simulink library "Lib_Turbo_Turbine_TMATS"  (R2012b)
settings: Solver=ode45  StartTime=0.0  StopTime=10.0  RelTol=1e-3
Description:
  | Thomas Modules
settings Model: Creator=jwchapm2  LastModifiedBy=jwchapm2

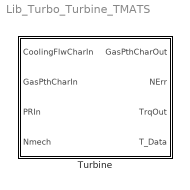
== system Lib_Turbo_Turbine_TMATS ==
  Turbine : Subsystem  mask(T-MATS: Turbine Library Block){X_T_PRVec_M=[ 3.000  8.000], Y_T_NcVec_M=[60 80  110], T_T_Map_WcArray_M=[0 0;0 0; 0 0], T_T_Map_EffArray_M=[0 0; 0 0; 0 0], s_T_Nc_M=0.0243, s_T_PR_M=0.9736, s_T_Wc_M=0.4504, s_T_Eff_M=0.9984, CFlwEn_M=off, T_CoolFlwPos_M=0, iDesign_M=off, NcDes_M=100, EffDes_M=0.9328, PRDes_M=5, NDes_M=10000}
      mask prompts: X_T_PRVec_M "X_T_PRVec_M - Turbine Map Pressure Ratio Vector (X-axis)(nx1)"; Y_T_NcVec_M "Y_T_NcVec_M - Turbine Map Corrected Speed Vector (Y-axis)(mx1)"; T_T_Map_WcArray_M "T_T_Map_WcArray_M - Turbine Map Flow Array (Wc=f(Nc,PR))(mxn)"; T_T_Map_EffArray_M "T_T_Map_EffArray_M - Turbine Map Efficiency Array (Eff = f(Nc,PR))(mxn)"; s_T_Nc_M "s_T_Nc_M - Corrected Speed Scalar Constant (T_Nc)"; s_T_PR_M "s_T_PR_M - Pressure Ratio Scalar Constant (T_PR)"; s_T_Wc_M "s_T_Wc_M - Flow Scalar Constant (T_Wc)"; s_T_Eff_M "s_T_Eff_M - Efficiency Scalar Constant (T_Eff)"; CFlwEn_M "CFlwEn_M - Cooling Flow Enable [0-off, 1-on]"; T_CoolFlwPos_M "T_CoolFlwPos_M - Cooling Flow position [0 at inlet,  1 at exit] (cx1)"; iDesign_M "iDesign_M - Calculate turbine map scalars based on design variables"; NcDes_M "NcDes_M - map Design Corrected Shaft Speed [rpm]"; EffDes_M "EffDes_M - Design Efficiency [frac]"; PRDes_M "PRDes_M - map Design Pressure Ratio [frac]"; NDes_M "NDes_M - Design Shaft Speed [rpm]"
      mask help: This block simulates the performance of a turbine using basic thermodynamic equations, properties, and table lookups.
      mask Help: web(which('Turbo_TMATS_Trb.html'),'-helpbrowser')
      mask Callback CFlwEn_M: MSK_SEC_Enables_TMATS('CFlwEn_M',10,'en')
      mask Callback iDesign_M:
      | MSK_SEC_Enables_TMATS('iDesign_M',[12 13 14 15],'en')
      | MSK_SEC_Enables_TMATS('iDesign_M',[5 6 7 8],'dis')

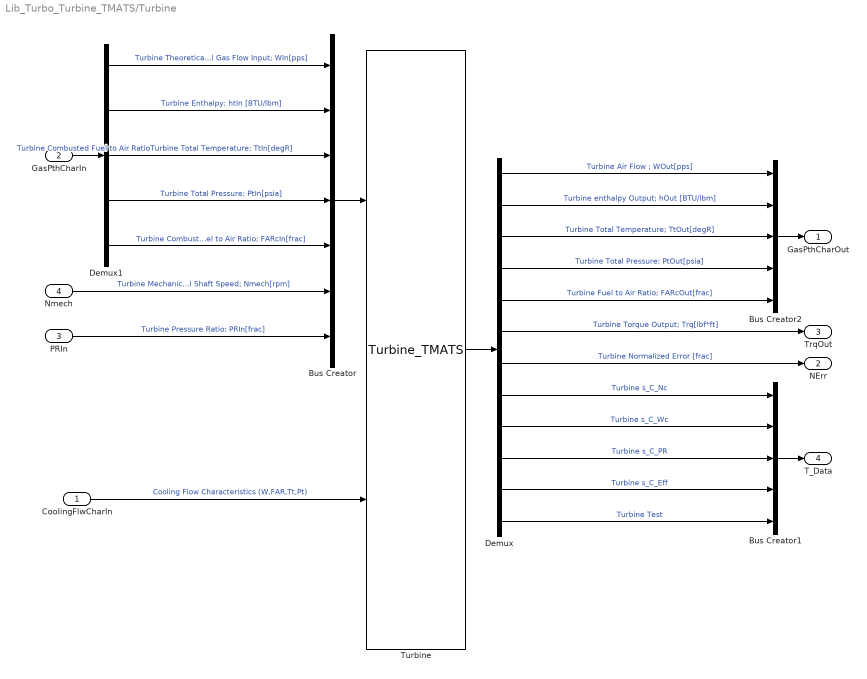
== system Lib_Turbo_Turbine_TMATS/Turbine ==
  CoolingFlwCharIn : Inport
  GasPthCharIn : Inport  Port=2
  PRIn : Inport  Port=3
  Nmech : Inport  Port=4
  Bus Creator : BusCreator  Inputs=7
  Bus Creator1 : BusCreator  Inputs=5
  Bus Creator2 : BusCreator  Inputs=5
  Demux : Demux  Outputs=12
  Demux1 : Demux  Outputs=5
  Turbine : S-Function  FunctionName=Turbine_TMATS  Parameters=s_T_Nc_M, s_T_PR_M, s_T_Wc_M, s_T_Eff_M, Y_T_NcVec_M, X_T_PRVec_M, T_T_Map_WcArray_M, T_T_Map_EffArray_M, T_CoolFlwPos_M, length(T_CoolFlwPos_M), CFlwEn_M, iDesign_M, NcDes_M, EffDes_M, PRDes_M, NDes_M, gcs  EnableBusSupport=off
  GasPthCharOut : Outport
  NErr : Outport  Port=2
  TrqOut : Outport  Port=3
  T_Data : Outport  Port=4
  wires:
  Demux/12 -> Bus Creator1/5  "Turbine Test"
  PRIn/1 -> Bus Creator/7  "Turbine Pressure Ratio; PRIn[frac]"
  Demux1/2 -> Bus Creator/2  "Turbine Enthalpy; htIn [BTU/lbm]"
  Demux1/3 -> Bus Creator/3  "Turbine Total Temperature; TtIn[degR]"
  Turbine/1 -> Demux/1
  Demux/1 -> Bus Creator2/1  "Turbine Air Flow ; WOut[pps]"
  Demux/5 -> Bus Creator2/5  "Turbine Fuel to Air Ratio; FARcOut[frac]"
  Demux/3 -> Bus Creator2/3  "Turbine Total Temperature; TtOut[degR]"
  Demux/4 -> Bus Creator2/4  "Turbine Total Pressure; PtOut[psia]"
  Bus Creator/1 -> Turbine/1
  Demux/2 -> Bus Creator2/2  "Turbine enthalpy Output; hOut [BTU/lbm]"
  Demux/6 -> TrqOut/1  "Turbine Torque Output; Trq[lbf*ft]"
  Nmech/1 -> Bus Creator/6  "Turbine Mechanical Shaft Speed; Nmech[rpm]"
  Demux1/4 -> Bus Creator/4  "Turbine Total Pressure; PtIn[psia]"
  Bus Creator2/1 -> GasPthCharOut/1
  GasPthCharIn/1 -> Demux1/1  "Turbine Combusted Fuel to Air Ratio"
  Demux1/1 -> Bus Creator/1  "Turbine Theoretical Gas Flow Input; WIn[pps]"
  Demux/7 -> NErr/1  "Turbine Normalized Error [frac]"
  CoolingFlwCharIn/1 -> Turbine/2  "Cooling Flow Characteristics (W,FAR,Tt,Pt)"
  Demux1/5 -> Bus Creator/5  "Turbine Combusted Fuel to Air Ratio; FARcIn[frac]"
  Bus Creator1/1 -> T_Data/1
  Demux/8 -> Bus Creator1/1  "Turbine s_C_Nc"
  Demux/9 -> Bus Creator1/2  "Turbine s_C_Wc"
  Demux/10 -> Bus Creator1/3  "Turbine s_C_PR"
  Demux/11 -> Bus Creator1/4  "Turbine s_C_Eff"
